simulink model "PMSM_ItscSat_Model_PriusMotor_InverseMap"  (R2024b)
settings: Solver=VariableStepAuto  StartTime=0.0  StopTime=0.03  FixedStep=1e-4
PostLoadFcn:
  | , if any(exist('dsrtsu_mdlpostloadfcn', 'file') == [2, 3, 6]), try dsrtsu_mdlpostloadfcn('Execute', bdroot); catch fprintf('Error in PostLoadFcn (dsrtsu_mdlpostloadfcn) for model "%s":\n %s\n', bdroot, lasterr); end, end,
undefined symbols (not defined in the file): ModelParam
libraries: simulink x1
PreSaveFcn:
  | , if any(exist('dsmpb_private', 'file') == [2, 3, 6]), try, dsmpb_private('dsmpb_mdlclblib', 'PreSave', bdroot); catch, disp(lasterr); end, end,
CloseFcn:
  | , if any(exist('dsmpb_private', 'file') == [2, 3, 6]), try, dsmpb_private('dsmpb_mdlclblib', 'Close', bdroot); catch, disp(lasterr); end, end,
settings Model: RTICANMMDATA=struct('GeneralSetupData',struct('modelroot','D:\01_XiL_SW\02_invhil-mlb_developer_3\ModuleTest','generalsettings',struct('filesettings',struct('destfolder',struct('Name','RTICANMM_FILES','Check',1),'buildfolder',struct('Name','.','Check',1),'AbsDestfolder',struct('Name','D:\01_XiL_SW\02_invhil-mlb_developer_3\ModuleTest\RTICANMM_FILES'),'AbsBuildfolder',struct('Name','D:\01_XiL_SW\02_invhil-mlb_developer_3\ModuleTest'))),'options',struct('addpaths',1,'rmpaths',1,'addtrcexclusion',logical(1),'cannavigator',struct('checkmonitoring',0),'show_usrtrc',0,'use_usrtrc',0),'advanced',struct('options',[1 1 1 1 1 1 1 1 1 1 1 1 1 1 1 1 1 1 1 1 1 1 1 1 1 1 1 1 1 1 1 1 1 1 1 1 1 1 1 1 1 1 1 1 1 1 1 1 1 1 1 1 1 1 1 1 1 1 1 1 1 1 1 1 1 1 1 1 1 1 1 1 1 1 1 1 1 1 1 1 1 1 1 1 1 1 1 1 1 1 1 1 1 1 1 1 1 1 1 1]),'MPSetup',{{}},'modelname','PMSM_Sat_Model_3ph_CrossSat_CT','block','PMSM_Sat_Model_3ph_CrossSat_CT'))  DSRTSU_INTERNAL_RTIFPGA=110  DSMPB_DATASERVER_ModelPortLibVersion1=8  DSMPB_DATASERVER_DataServerVersion1=6  DSMPB_DATASERVER_DataServerStreamVersion1=3  Creator=jkoupeny  LastModifiedBy=Tulajdonos
settings SolverCC: AlgebraicLoopSolver=TrustRegion
settings DataIOCC: ReturnWorkspaceOutputs=off
settings OptimizationCC: EfficientMapNaN2IntZero=off
settings DebuggingCC: UnconnectedInputMsg=warning  UnconnectedOutputMsg=warning  UnconnectedLineMsg=warning  ArithmeticOperatorsInVariantConditions=warning
settings HardwareCC: TargetBitPerPointer=64  TargetBitPerSizeT=64  TargetBitPerPtrDiffT=64  TargetLongLongMode=on  TargetIntDivRoundTo=Zero  TargetEndianess=LittleEndian  TargetWordSize=64  TargetHWDeviceType=MATLAB Host  ProdEqTarget=off
settings ModelReferenceCC: EnableRefExpFcnMdlSchedulingChecks=on
settings SFSimCC: SimUseLocalCustomCode=off  CustomCodeUndefinedFunction=UseInterfaceOnly
settings RTWCC: RTWUseLocalCustomCode=off  GPUComputeCapability=3.5
settings CodeAppCC: MaxIdLength=128  StateflowObjectComments=on
settings GRTTargetCC: TargetLangStandard=C89/C90 (ANSI)  CombineOutputUpdateFcns=off  GRTInterface=on

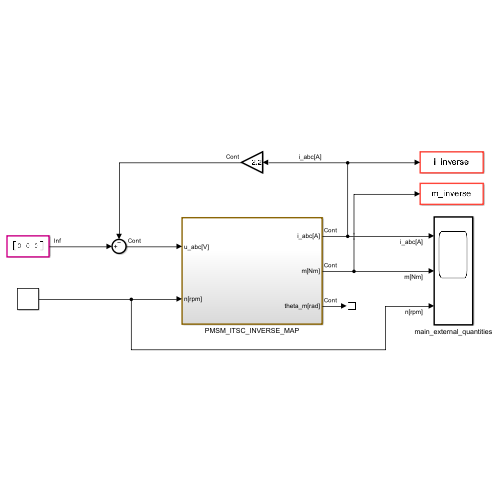
[thumbnail: Simulink's stored preview of the top-level diagram]
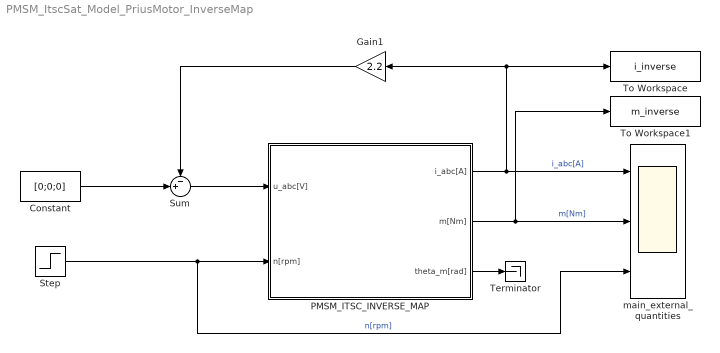
== system PMSM_ItscSat_Model_PriusMotor_InverseMap ==
  Constant : Constant  Value=[0;0;0]
  Gain1 : Gain  Gain=2.2
  PMSM_ITSC_INVERSE_MAP : Subsystem
  Step : Step  Time=0  After=2500  SampleTime=0
  Sum : Sum  Inputs=-+|
  Terminator : Terminator
  To Workspace : ToWorkspace  VariableName=i_inverse  SaveFormat=Timeseries  SampleTime=1e-4
  To Workspace1 : ToWorkspace  VariableName=m_inverse  SaveFormat=Timeseries  SampleTime=1e-4
  main_external_quantities : Scope  NumInputPorts=3
  wires:
  PMSM_ITSC_INVERSE_MAP/2(m[Nm]) -> To Workspace1/1, main_external_quantities/2  "m[Nm]"
  PMSM_ITSC_INVERSE_MAP/3(theta_m[rad]) -> Terminator/1
  Step/1 -> main_external_quantities/3, PMSM_ITSC_INVERSE_MAP/2(n[rpm])  "n[rpm]"
  PMSM_ITSC_INVERSE_MAP/1(i_abc[A]) -> Gain1/1, To Workspace/1, main_external_quantities/1  "i_abc[A]"
  Sum/1 -> PMSM_ITSC_INVERSE_MAP/1(u_abc[V])
  Constant/1 -> Sum/2
  Gain1/1 -> Sum/1

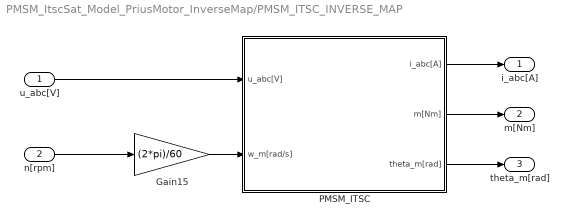
== system PMSM_ItscSat_Model_PriusMotor_InverseMap/PMSM_ITSC_INVERSE_MAP ==
  u_abc[V] : Inport
  n[rpm] : Inport  Port=2
  Gain15 : Gain  Gain=(2*pi)/60
  PMSM_ITSC : Subsystem
  i_abc[A] : Outport
  m[Nm] : Outport  Port=2
  theta_m[rad] : Outport  Port=3
  wires:
  n[rpm]/1 -> Gain15/1
  Gain15/1 -> PMSM_ITSC/2(w_m[rad/s])
  PMSM_ITSC/2(m[Nm]) -> m[Nm]/1
  PMSM_ITSC/3(theta_m[rad]) -> theta_m[rad]/1
  PMSM_ITSC/1(i_abc[A]) -> i_abc[A]/1
  u_abc[V]/1 -> PMSM_ITSC/1(u_abc[V])

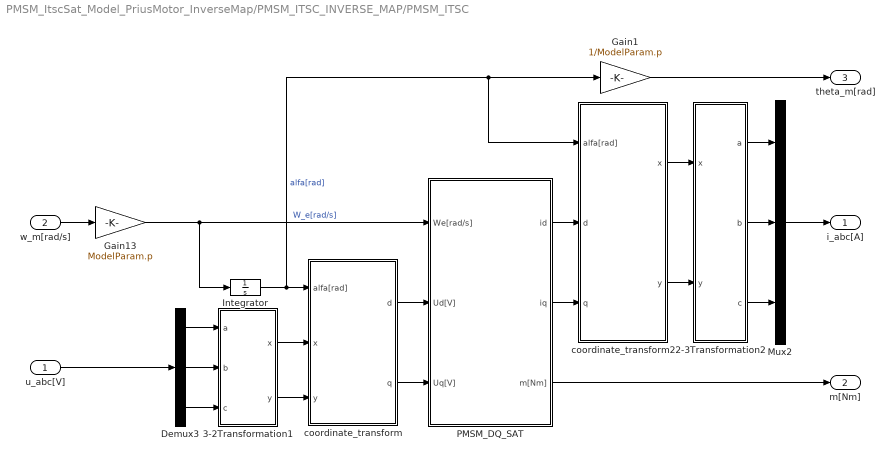
== system PMSM_ItscSat_Model_PriusMotor_InverseMap/PMSM_ITSC_INVERSE_MAP/PMSM_ITSC ==
  u_abc[V] : Inport
  w_m[rad/s] : Inport  Port=2
  2-3Transformation2 : Subsystem
  3-2Transformation1 : Subsystem
  Demux3 : Demux  Outputs=3
  Gain1 : Gain  Gain=1/ModelParam.p
  Gain13 : Gain  Gain=ModelParam.p
  Integrator : Integrator
  Mux2 : Mux  Inputs=3
  PMSM_DQ_SAT : Subsystem
  coordinate_transform : Subsystem
  coordinate_transform2 : Subsystem
  i_abc[A] : Outport
  m[Nm] : Outport  Port=2
  theta_m[rad] : Outport  Port=3
  wires:
  2-3Transformation2/1(a) -> Mux2/1
  Gain1/1 -> theta_m[rad]/1
  w_m[rad/s]/1 -> Gain13/1
  Gain13/1 -> Integrator/1, PMSM_DQ_SAT/1(We[rad/s])  "W_e[rad/s]"
  u_abc[V]/1 -> Demux3/1
  3-2Transformation1/2(y) -> coordinate_transform/3(y)
  3-2Transformation1/1(x) -> coordinate_transform/2(x)
  coordinate_transform/2(q) -> PMSM_DQ_SAT/3(Uq[V])
  coordinate_transform/1(d) -> PMSM_DQ_SAT/2(Ud[V])
  Demux3/2 -> 3-2Transformation1/2(b)
  Demux3/1 -> 3-2Transformation1/1(a)
  Demux3/3 -> 3-2Transformation1/3(c)
  PMSM_DQ_SAT/2(iq) -> coordinate_transform2/3(q)
  PMSM_DQ_SAT/1(id) -> coordinate_transform2/2(d)
  Integrator/1 -> coordinate_transform2/1(alfa[rad]), Gain1/1, coordinate_transform/1(alfa[rad])  "alfa[rad]"
  coordinate_transform2/2(y) -> 2-3Transformation2/2(y)
  coordinate_transform2/1(x) -> 2-3Transformation2/1(x)
  Mux2/1 -> i_abc[A]/1
  2-3Transformation2/2(b) -> Mux2/2
  2-3Transformation2/3(c) -> Mux2/3
  PMSM_DQ_SAT/3(m[Nm]) -> m[Nm]/1

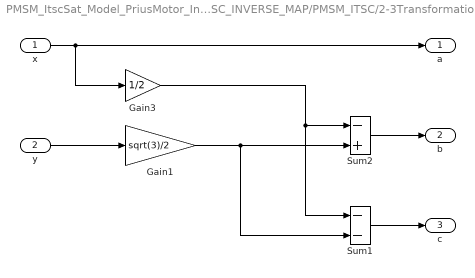
== system PMSM_ItscSat_Model_PriusMotor_InverseMap/PMSM_ITSC_INVERSE_MAP/PMSM_ITSC/2-3Transformation2 ==
  x : Inport
  y : Inport  Port=2
  Gain1 : Gain  Gain=sqrt(3)/2  SaturateOnIntegerOverflow=on  OutDataTypeStr=Inherit: Same as input  ParamDataTypeStr=Inherit: Same as input
  Gain3 : Gain  Gain=1/2  SaturateOnIntegerOverflow=on  OutDataTypeStr=Inherit: Same as input  ParamDataTypeStr=Inherit: Same as input
  Sum1 : Sum  Inputs=--  InputSameDT=on  SaturateOnIntegerOverflow=on  OutDataTypeStr=Inherit: Same as first input
  Sum2 : Sum  Inputs=-+  InputSameDT=on  SaturateOnIntegerOverflow=on  OutDataTypeStr=Inherit: Same as first input
  a : Outport
  b : Outport  Port=2
  c : Outport  Port=3
  wires:
  Gain3/1 -> Sum2/1, Sum1/1
  Gain1/1 -> Sum1/2, Sum2/2
  x/1 -> Gain3/1, a/1
  Sum1/1 -> c/1
  y/1 -> Gain1/1
  Sum2/1 -> b/1

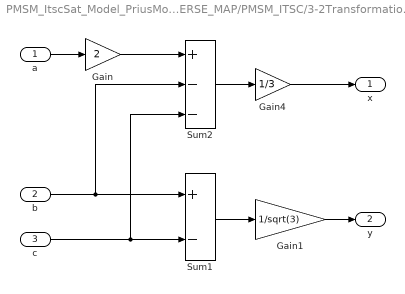
== system PMSM_ItscSat_Model_PriusMotor_InverseMap/PMSM_ITSC_INVERSE_MAP/PMSM_ITSC/3-2Transformation1 ==
  a : Inport
  b : Inport  Port=2
  c : Inport  Port=3
  Gain : Gain  Gain=2  SaturateOnIntegerOverflow=on  OutDataTypeStr=Inherit: Same as input  ParamDataTypeStr=Inherit: Same as input
  Gain1 : Gain  Gain=1/sqrt(3)  SaturateOnIntegerOverflow=on  OutDataTypeStr=Inherit: Same as input  ParamDataTypeStr=Inherit: Same as input
  Gain4 : Gain  Gain=1/3  SaturateOnIntegerOverflow=on  OutDataTypeStr=Inherit: Same as input  ParamDataTypeStr=Inherit: Same as input
  Sum1 : Sum  Inputs=+-  InputSameDT=on  SaturateOnIntegerOverflow=on  OutDataTypeStr=Inherit: Same as first input
  Sum2 : Sum  Inputs=+--  InputSameDT=on  SaturateOnIntegerOverflow=on  OutDataTypeStr=Inherit: Same as first input
  x : Outport
  y : Outport  Port=2
  wires:
  a/1 -> Gain/1
  Sum1/1 -> Gain1/1
  Gain1/1 -> y/1
  b/1 -> Sum1/1, Sum2/2
  c/1 -> Sum1/2, Sum2/3
  Gain/1 -> Sum2/1
  Sum2/1 -> Gain4/1
  Gain4/1 -> x/1

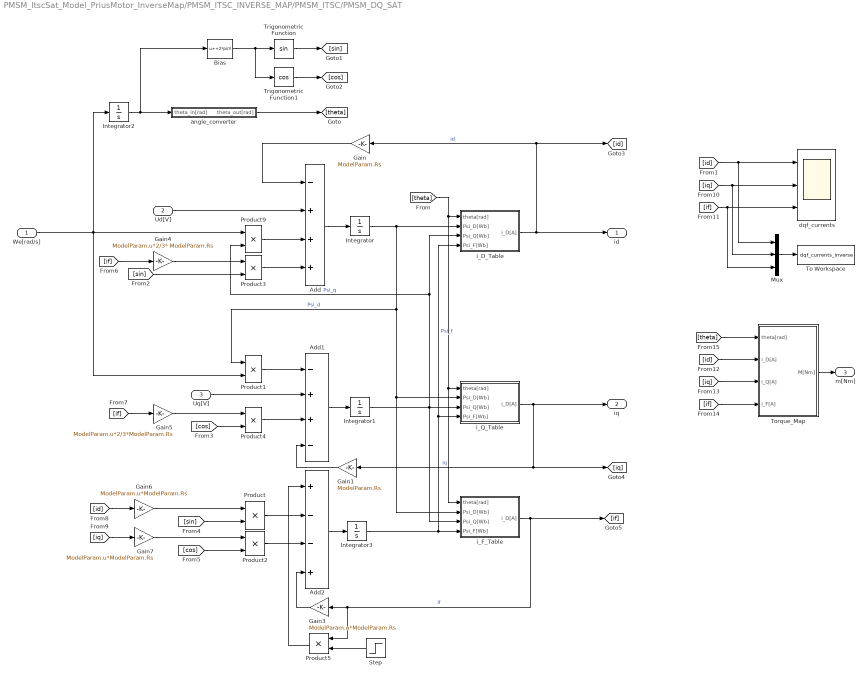
== system PMSM_ItscSat_Model_PriusMotor_InverseMap/PMSM_ITSC_INVERSE_MAP/PMSM_ITSC/PMSM_DQ_SAT ==
  We[rad/s] : Inport
  Ud[V] : Inport  Port=2
  Uq[V] : Inport  Port=3
  Add : Sum  Inputs=-+++
  Add1 : Sum  Inputs=-++-
  Add2 : Sum  Inputs=+--+
  Bias : Bias  Bias=+2*pi/3  SaturateOnIntegerOverflow=off
  Gain : Gain  Gain=ModelParam.Rs
  Gain1 : Gain  Gain=ModelParam.Rs
  Gain3 : Gain  Gain=ModelParam.u*ModelParam.Rs
  Gain4 : Gain  Gain=ModelParam.u*2/3* ModelParam.Rs
  Gain5 : Gain  Gain=ModelParam.u*2/3*ModelParam.Rs
  Gain6 : Gain  Gain=ModelParam.u*ModelParam.Rs
  Gain7 : Gain  Gain=ModelParam.u*ModelParam.Rs
  Integrator : Integrator  InitialCondition=ModelParam.MachineModel.PsidInit
  Integrator1 : Integrator  InitialCondition=ModelParam.MachineModel.PsiqInit
  Integrator2 : Integrator
  Integrator3 : Integrator  InitialCondition=ModelParam.MachineModel.PsifInit
  Mux : Mux  Inputs=3
  Product : Product
  Product{1,3..4,9} (4 alike) : Product  RndMeth=Zero
  Product2 : Product
  Product5 : Product
  Step : Step  Time=0.015  Before=ModelParam.Rf  After=ModelParam.Rf/10  SampleTime=0
  To Workspace : ToWorkspace  VariableName=dqf_currents_inverse  SaveFormat=Timeseries  SampleTime=1e-4
  Torque_Map : Subsystem
  Trigonometric Function : Trigonometry
  Trigonometric Function1 : Trigonometry  Operator=cos
  angle_converter : Subsystem
  dqf_currents : Scope  NumInputPorts=3
  i_D_Table : Subsystem
  i_F_Table : Subsystem
  i_Q_Table : Subsystem
  id : Outport
  iq : Outport  Port=2
  m[Nm] : Outport  Port=3
  wires:
  Add1/1 -> Integrator1/1
  Uq[V]/1 -> Add1/2
  Ud[V]/1 -> Add/2
  Add/1 -> Integrator/1
  We[rad/s]/1 -> Product1/2, Integrator2/1, Product9/1
  i_D_Table/1(i_D[A]) -> id/1, [id], Gain/1  "id"
  Integrator/1 -> i_D_Table/2(Psi_D[Wb]), i_F_Table/2(Psi_D[Wb]), i_Q_Table/2(Psi_D[Wb]), Product1/1  "Psi_d"
  Integrator1/1 -> i_F_Table/3(Psi_Q[Wb]), i_Q_Table/3(Psi_Q[Wb]), i_D_Table/3(Psi_Q[Wb]), Product9/2  "Psi_q"
  Gain/1 -> Add/1
  Gain1/1 -> Add1/4
  Torque_Map/1(M[Nm]) -> m[Nm]/1
  Product9/1 -> Add/3
  Product1/1 -> Add1/1
  Add2/1 -> Integrator3/1
  Integrator3/1 -> i_F_Table/4(Psi_F[Wb]), i_Q_Table/4(Psi_F[Wb]), i_D_Table/4(Psi_F[Wb])  "Psi_f"
  angle_converter/1(theta_out[rad]) -> [theta]
  [theta] -> i_F_Table/1(theta[rad]), i_Q_Table/1(theta[rad]), i_D_Table/1(theta[rad])
  i_Q_Table/1(i_D[A]) -> Gain1/1, [iq], iq/1  "iq"
  i_F_Table/1(i_D[A]) -> [if], Product5/1, Gain3/1  "if"
  Integrator2/1 -> Bias/1, angle_converter/1(theta_in[rad])
  Trigonometric Function/1 -> [sin]
  Trigonometric Function1/1 -> [cos]
  Product/1 -> Add2/2
  Product2/1 -> Add2/3
  [sin] -> Product/2
  [cos] -> Product2/2
  Product5/1 -> Add2/1
  Gain3/1 -> Add2/4
  [if] -> Gain4/1
  Product3/1 -> Add/4
  Gain4/1 -> Product3/1
  [sin] -> Product3/2
  Product4/1 -> Add1/3
  [if] -> Gain5/1
  Gain5/1 -> Product4/1
  [cos] -> Product4/2
  [id] -> Gain6/1
  [iq] -> Gain7/1
  Gain7/1 -> Product2/1
  Gain6/1 -> Product/1
  Bias/1 -> Trigonometric Function1/1, Trigonometric Function/1
  Step/1 -> Product5/2
  [id] -> Mux/1, dqf_currents/1
  [iq] -> Mux/2, dqf_currents/2
  [if] -> Mux/3, dqf_currents/3
  [id] -> Torque_Map/2(i_D[A])
  [iq] -> Torque_Map/3(i_Q[A])
  [if] -> Torque_Map/4(i_F[A])
  [theta] -> Torque_Map/1(theta[rad])
  Mux/1 -> To Workspace/1

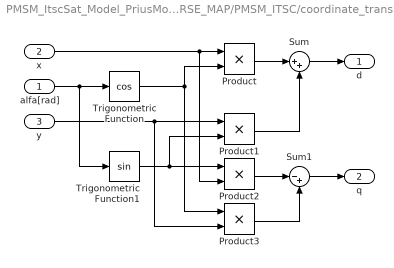
== system PMSM_ItscSat_Model_PriusMotor_InverseMap/PMSM_ITSC_INVERSE_MAP/PMSM_ITSC/coordinate_transform ==
  alfa[rad] : Inport
  x : Inport  Port=2
  y : Inport  Port=3
  Product{,1..3} (4 alike) : Product  RndMeth=Zero
  Sum : Sum  Inputs=|++
  Sum1 : Sum  Inputs=|-+
  Trigonometric Function : Trigonometry  Operator=cos
  Trigonometric Function1 : Trigonometry
  d : Outport
  q : Outport  Port=2
  wires:
  x/1 -> Product/1, Product2/2
  alfa[rad]/1 -> Trigonometric Function/1, Trigonometric Function1/1
  Product/1 -> Sum/1
  Product1/1 -> Sum/2
  Sum/1 -> d/1
  Trigonometric Function/1 -> Product/2, Product3/1
  y/1 -> Product1/1, Product3/2
  Trigonometric Function1/1 -> Product1/2, Product2/1
  Product2/1 -> Sum1/1
  Product3/1 -> Sum1/2
  Sum1/1 -> q/1

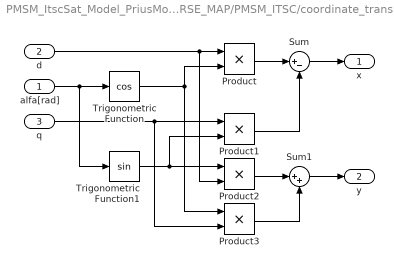
== system PMSM_ItscSat_Model_PriusMotor_InverseMap/PMSM_ITSC_INVERSE_MAP/PMSM_ITSC/coordinate_transform2 ==
  alfa[rad] : Inport
  d : Inport  Port=2
  q : Inport  Port=3
  Product{,1..3} (4 alike) : Product  RndMeth=Zero
  Sum : Sum  Inputs=|+-
  Sum1 : Sum  Inputs=|++
  Trigonometric Function : Trigonometry  Operator=cos
  Trigonometric Function1 : Trigonometry
  x : Outport
  y : Outport  Port=2
  wires:
  Sum1/1 -> y/1
  Product3/1 -> Sum1/2
  Product2/1 -> Sum1/1
  Trigonometric Function1/1 -> Product2/1, Product1/2
  q/1 -> Product3/2, Product1/1
  Trigonometric Function/1 -> Product3/1, Product/2
  Sum/1 -> x/1
  Product1/1 -> Sum/2
  Product/1 -> Sum/1
  alfa[rad]/1 -> Trigonometric Function1/1, Trigonometric Function/1
  d/1 -> Product2/2, Product/1

== system PMSM_ItscSat_Model_PriusMotor_InverseMap/PMSM_ITSC_INVERSE_MAP/PMSM_ITSC/PMSM_DQ_SAT/Torque_Map ==
  theta[rad] : Inport
  i_D[A] : Inport  Port=2
  i_Q[A] : Inport  Port=3
  i_F[A] : Inport  Port=4
  4-D Lookup Table : Lookup_n-D  NumberOfTableDimensions=4  BreakpointsForDimension1=ModelParam.MachineModel.IdGrid  BreakpointsForDimension2=ModelParam.MachineModel.IqGrid  BreakpointsForDimension3=ModelParam.MachineModel.IfGrid  BreakpointsForDimension4=ModelParam.MachineModel.ThetaGrid  Table=ModelParam.MachineModel.TorqueMap  InterpMethod=Cubic spline  InternalRulePriority=Speed  RndMeth=Simplest
      settings: InputPortMap=u0,u1,u2,u3
  M[Nm] : Outport
  wires:
  i_F[A]/1 -> 4-D Lookup Table/3
  theta[rad]/1 -> 4-D Lookup Table/4
  4-D Lookup Table/1 -> M[Nm]/1
  i_Q[A]/1 -> 4-D Lookup Table/2
  i_D[A]/1 -> 4-D Lookup Table/1

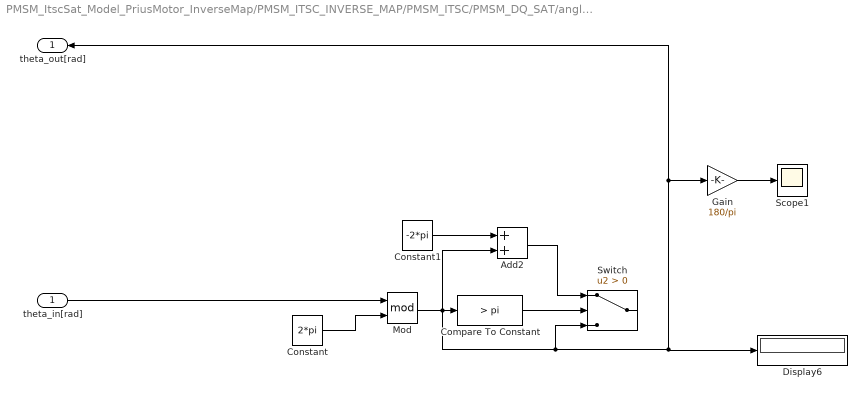
== system PMSM_ItscSat_Model_PriusMotor_InverseMap/PMSM_ITSC_INVERSE_MAP/PMSM_ITSC/PMSM_DQ_SAT/angle_converter ==
  theta_in[rad] : Inport
  Add2 : Sum
  Compare To Constant : simulink/Logic and Bit Operations/Compare To Constant  relop=>  const=pi  OutDataTypeStr=boolean  ZeroCross=off
  Constant : Constant  Value=2*pi
  Constant1 : Constant  Value=-2*pi
  Display6 : Display
  Gain : Gain  Gain=180/pi
  Mod : Math  Operator=mod
  Scope1 : Scope
  Switch : Switch  Criteria=u2 > Threshold  SaturateOnIntegerOverflow=off  InputSameDT=off
  theta_out[rad] : Outport
  wires:
  Mod/1 -> Add2/2, Display6/1, theta_out[rad]/1, Gain/1, Switch/3, Compare To Constant/1
  Constant1/1 -> Add2/1
  Constant/1 -> Mod/2
  Compare To Constant/1 -> Switch/2
  Add2/1 -> Switch/1
  theta_in[rad]/1 -> Mod/1
  Gain/1 -> Scope1/1

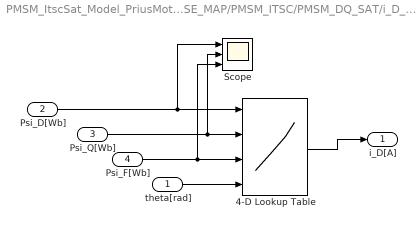
== system PMSM_ItscSat_Model_PriusMotor_InverseMap/PMSM_ITSC_INVERSE_MAP/PMSM_ITSC/PMSM_DQ_SAT/i_D_Table ==
  theta[rad] : Inport
  Psi_D[Wb] : Inport  Port=2
  Psi_Q[Wb] : Inport  Port=3
  Psi_F[Wb] : Inport  Port=4
  4-D Lookup Table : Lookup_n-D  NumberOfTableDimensions=4  BreakpointsForDimension1=ModelParam.MachineModel.PsidGrid  BreakpointsForDimension2=ModelParam.MachineModel.PsiqGrid  BreakpointsForDimension3=ModelParam.MachineModel.PsifGrid  BreakpointsForDimension4=ModelParam.MachineModel.ThetaGrid  Table=ModelParam.MachineModel.IdMap  InterpMethod=Cubic spline  InternalRulePriority=Speed  RndMeth=Simplest
      settings: InputPortMap=u0,u1,u2,u3
  Scope : Scope  NumInputPorts=3
  i_D[A] : Outport
  wires:
  Psi_D[Wb]/1 -> Scope/1, 4-D Lookup Table/1
  Psi_Q[Wb]/1 -> Scope/2, 4-D Lookup Table/2
  4-D Lookup Table/1 -> i_D[A]/1
  theta[rad]/1 -> 4-D Lookup Table/4
  Psi_F[Wb]/1 -> Scope/3, 4-D Lookup Table/3

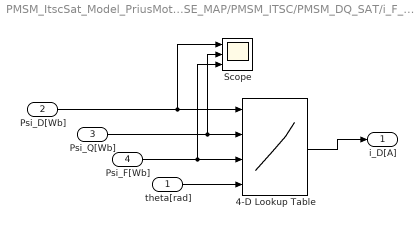
== system PMSM_ItscSat_Model_PriusMotor_InverseMap/PMSM_ITSC_INVERSE_MAP/PMSM_ITSC/PMSM_DQ_SAT/i_F_Table ==
  theta[rad] : Inport
  Psi_D[Wb] : Inport  Port=2
  Psi_Q[Wb] : Inport  Port=3
  Psi_F[Wb] : Inport  Port=4
  4-D Lookup Table : Lookup_n-D  NumberOfTableDimensions=4  BreakpointsForDimension1=ModelParam.MachineModel.PsidGrid  BreakpointsForDimension2=ModelParam.MachineModel.PsiqGrid  BreakpointsForDimension3=ModelParam.MachineModel.PsifGrid  BreakpointsForDimension4=ModelParam.MachineModel.ThetaGrid  Table=ModelParam.MachineModel.IfMap  InterpMethod=Cubic spline  InternalRulePriority=Speed  RndMeth=Simplest
      settings: InputPortMap=u0,u1,u2,u3
  Scope : Scope  NumInputPorts=3
  i_D[A] : Outport
  wires:
  Psi_D[Wb]/1 -> Scope/1, 4-D Lookup Table/1
  Psi_Q[Wb]/1 -> Scope/2, 4-D Lookup Table/2
  4-D Lookup Table/1 -> i_D[A]/1
  theta[rad]/1 -> 4-D Lookup Table/4
  Psi_F[Wb]/1 -> Scope/3, 4-D Lookup Table/3

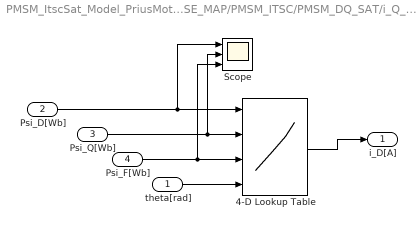
== system PMSM_ItscSat_Model_PriusMotor_InverseMap/PMSM_ITSC_INVERSE_MAP/PMSM_ITSC/PMSM_DQ_SAT/i_Q_Table ==
  theta[rad] : Inport
  Psi_D[Wb] : Inport  Port=2
  Psi_Q[Wb] : Inport  Port=3
  Psi_F[Wb] : Inport  Port=4
  4-D Lookup Table : Lookup_n-D  NumberOfTableDimensions=4  BreakpointsForDimension1=ModelParam.MachineModel.PsidGrid  BreakpointsForDimension2=ModelParam.MachineModel.PsiqGrid  BreakpointsForDimension3=ModelParam.MachineModel.PsifGrid  BreakpointsForDimension4=ModelParam.MachineModel.ThetaGrid  Table=ModelParam.MachineModel.IqMap  InterpMethod=Cubic spline  InternalRulePriority=Speed  RndMeth=Simplest
      settings: InputPortMap=u0,u1,u2,u3
  Scope : Scope  NumInputPorts=3
  i_D[A] : Outport
  wires:
  Psi_F[Wb]/1 -> 4-D Lookup Table/3, Scope/3
  theta[rad]/1 -> 4-D Lookup Table/4
  4-D Lookup Table/1 -> i_D[A]/1
  Psi_Q[Wb]/1 -> 4-D Lookup Table/2, Scope/2
  Psi_D[Wb]/1 -> 4-D Lookup Table/1, Scope/1
